simulink model "EulerKinematicalEquations"  (R2023b)
settings: Solver=FixedStepAuto  StartTime=0.0  StopTime=100  FixedStep=.05  RelTol=1e-3
values from neighbouring files (symbols this model uses):
  q0 = angle2quat(phidot,thetadot,psidot)    [F4ModelCode.m]    (also in F4ModelCodeV2.m; F4ModelCodeV2Q2PartD.m)
undefined symbols (not defined in the file or in its folder): phi0, psi0, theta0
settings Model: Creator=Christopher  LastModifiedBy=Owner
settings SolverCC: AlgebraicLoopSolver=TrustRegion
settings DataIOCC: ReturnWorkspaceOutputs=off
settings DebuggingCC: UnconnectedInputMsg=warning  UnconnectedOutputMsg=warning  UnconnectedLineMsg=warning  ArithmeticOperatorsInVariantConditions=warning
settings ModelReferenceCC: EnableRefExpFcnMdlSchedulingChecks=on
settings SFSimCC: CustomCodeUndefinedFunction=UseInterfaceOnly
settings RTWCC: DLArmComputeVersion=19.05

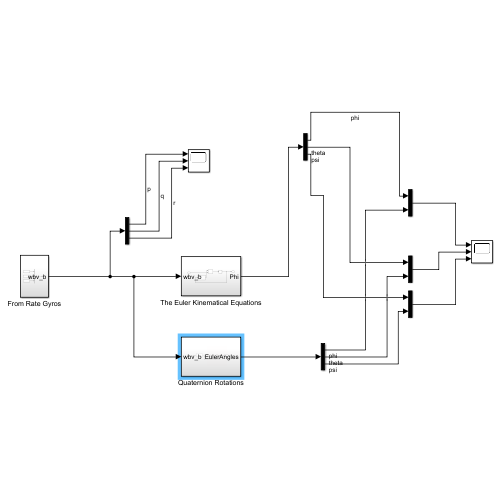
[thumbnail: Simulink's stored preview of the top-level diagram]
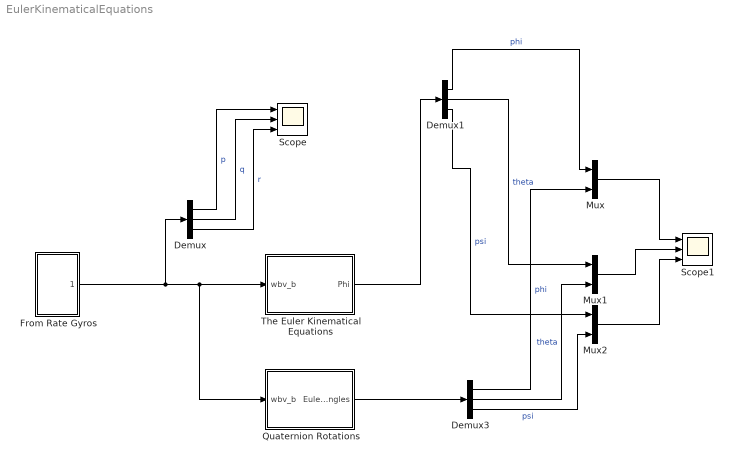
== system EulerKinematicalEquations ==
  Demux : Demux  Outputs=3
  Demux1 : Demux  Outputs=3
  Demux3 : Demux  Outputs=3
  From Rate Gyros : Subsystem
  Mux : Mux  Inputs=2
  Mux1 : Mux  Inputs=2
  Mux2 : Mux  Inputs=2
  Quaternion Rotations : Subsystem
  Scope : Scope  NumInputPorts=3
  Scope1 : Scope  NumInputPorts=3
  The Euler Kinematical Equations : Subsystem
  wires:
  From Rate Gyros/1(wbv_b) -> Demux/1, Quaternion Rotations/1(wbv_b), The Euler Kinematical Equations/1(wbv_b)
  Demux/1 -> Scope/1  "p"
  Demux/2 -> Scope/2  "q"
  Demux/3 -> Scope/3  "r"
  Demux1/2 -> Mux1/1  "theta"
  Demux1/1 -> Mux/1  "phi"
  The Euler Kinematical Equations/1(Phi) -> Demux1/1
  Mux/1 -> Scope1/1
  Mux1/1 -> Scope1/2
  Mux2/1 -> Scope1/3
  Quaternion Rotations/1(EulerAngles) -> Demux3/1
  Demux3/1 -> Mux/2  "phi"
  Demux1/3 -> Mux2/1  "psi"
  Demux3/2 -> Mux1/2  "theta"
  Demux3/3 -> Mux2/2  "psi"

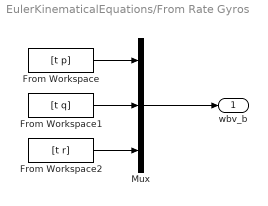
== system EulerKinematicalEquations/From Rate Gyros ==
  From Workspace : FromWorkspace  VariableName=[t p]
  From Workspace1 : FromWorkspace  VariableName=[t q]
  From Workspace2 : FromWorkspace  VariableName=[t r]
  Mux : Mux  Inputs=3
  wbv_b : Outport  VectorParamsAs1DForOutWhenUnconnected=off
  wires:
  From Workspace/1 -> Mux/1
  From Workspace1/1 -> Mux/2
  Mux/1 -> wbv_b/1
  From Workspace2/1 -> Mux/3

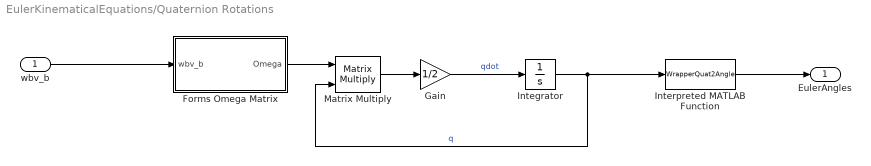
== system EulerKinematicalEquations/Quaternion Rotations ==
  wbv_b : Inport
  Forms Omega Matrix : MATLAB Function  TreatAsAtomicUnit=on
  Gain : Gain  Gain=1/2
  Integrator : Integrator  InitialCondition=q0
  Interpreted MATLAB Function : MATLABFcn  MATLABFcn=WrapperQuat2Angle
  Matrix Multiply : Product  Multiplication=Matrix(*)
  EulerAngles : Outport  VectorParamsAs1DForOutWhenUnconnected=off
  wires:
  Gain/1 -> Integrator/1  "qdot"
  Interpreted MATLAB Function/1 -> EulerAngles/1
  Integrator/1 -> Interpreted MATLAB Function/1, Matrix Multiply/2  "q"
  Matrix Multiply/1 -> Gain/1
  wbv_b/1 -> Forms Omega Matrix/1(wbv_b)
  Forms Omega Matrix/1(Omega) -> Matrix Multiply/1

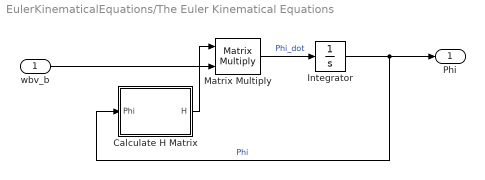
== system EulerKinematicalEquations/The Euler Kinematical Equations ==
  wbv_b : Inport
  Calculate H Matrix : MATLAB Function  TreatAsAtomicUnit=on
  Integrator : Integrator  InitialCondition=[phi0;theta0;psi0]
  Matrix Multiply : Product  Multiplication=Matrix(*)
  Phi : Outport  VectorParamsAs1DForOutWhenUnconnected=off
  wires:
  Integrator/1 -> Phi/1, Calculate H Matrix/1(Phi)  "Phi"
  Matrix Multiply/1 -> Integrator/1  "Phi_dot"
  wbv_b/1 -> Matrix Multiply/2
  Calculate H Matrix/1(H) -> Matrix Multiply/1

== matlab function EulerKinematicalEquations/Quaternion Rotations/Forms Omega Matrix ==
  data: wbv_b input; Omega output
function Omega  = fcn(wbv_b)

wx = wbv_b(1);
wy = wbv_b(2);
wz = wbv_b(3);

Omega = [0 -wx -wy -wz;
    wx 0 wz -wy;
    wy -wz 0 wx;
    wz wy -wx 0];

== matlab function EulerKinematicalEquations/The Euler Kinematical Equations/Calculate H Matrix ==
  data: Phi input; H output
function H = fcn(Phi)

%Unpack Phi
phi     = Phi(1);
theta   = Phi(2);
psi     = Phi(3);

%Input the H matrix
H = [1 tan(theta)*sin(phi) tan(theta)*cos(phi);
    0 cos(phi) -sin(phi);
    0 sin(phi)/cos(theta) cos(phi)/cos(theta)];
